simulink model "GonzalezGC21210380P3LC"  (R2024b)
settings: Solver=ode15s  StartTime=0.0  StopTime=10  MaxStep=1E-3  RelTol=1e-3
libraries: slpidlib x1
settings DataIOCC: ReturnWorkspaceOutputs=off  TimeSaveName=t
settings DebuggingCC: AlgebraicLoopMsg=none  ArtificialAlgebraicLoopMsg=none  BlockPriorityViolationMsg=error  MinStepSizeMsg=error  MaxConsecutiveZCsMsg=none  OperatingPointInterfaceChecksumMismatchMsg=none

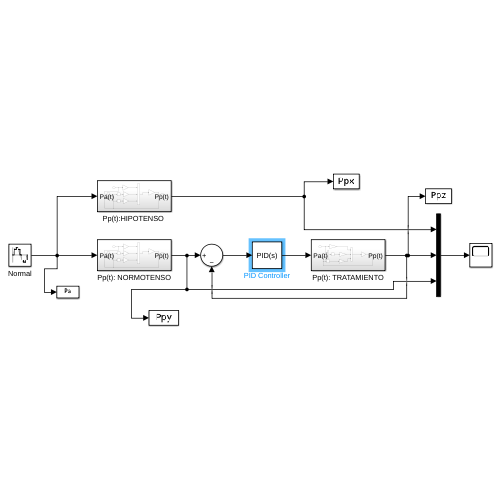
[thumbnail: Simulink's stored preview of the top-level diagram]
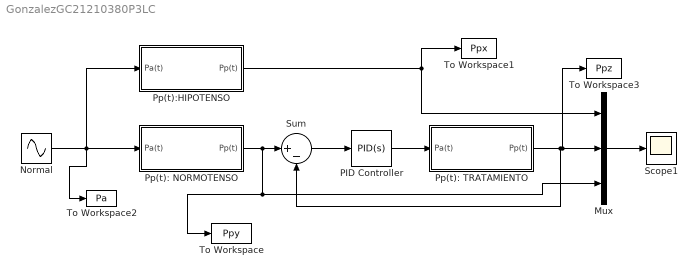
== system GonzalezGC21210380P3LC ==
  Mux : Mux  Inputs=3
  Normal : Sin  Bias=0.8  Frequency=(2*pi)*(95/60)  SampleTime=0.001
  PID Controller : slpidlib/PID Controller  Controller=PID  Form=Parallel  TimeDomain=Continuous-time  UseExternalTs=off  SampleTime=-1  IntegratorMethod=Forward Euler  FilterMethod=Forward Euler  ControllerParametersSource=internal  P=0  I=551.4981  UseKiTs=off  D=0  UseExternalDerivativeSource=off  N=100  UseFilter=on  TunerSelectOption=Transfer Function Based (PID Tuner App)  InitialConditionSource=internal  InitialConditionForIntegrator=0  InitialConditionForFilter=0  DifferentiatorICPrevScaledInput=0  ExternalReset=none  TrackingMode=off  Kt=1  LimitOutput=off  SatLimitsSource=internal  UpperSaturationLimit=inf  LowerSaturationLimit=-inf  LinearizeAsGain=on  AntiWindupMode=none  Kb=1  LimitIntegrator=off  UpperIntegratorSaturationLimit=inf  LowerIntegratorSaturationLimit=-inf  POutMin=[]  POutMax=[]  IOutMin=[]  IOutMax=[]  DOutMin=[]  DOutMax=[]  NOutMin=[]  NOutMax=[]  SumOutMin=[]  SumOutMax=[]  SaturationOutMin=[]  SaturationOutMax=[]  PParamMin=[]  PParamMax=[]  IParamMin=[]  IParamMax=[]  DParamMin=[]  DParamMax=[]  NParamMin=[]  NParamMax=[]  KbParamMin=[]  KbParamMax=[]  KtParamMin=[]  KtParamMax=[]  KbOutMin=[]  KbOutMax=[]  KtOutMin=[]  KtOutMax=[]  IntegratorOutMin=[]  IntegratorOutMax=[]  FilterOutMin=[]  FilterOutMax=[]  SumI1OutMin=[]  SumI1OutMax=[]  SumI2OutMin=[]  SumI2OutMax=[]  SumI3OutMin=[]  SumI3OutMax=[]  SumI4OutMin=[]  SumI4OutMax=[]  SumDOutMin=[]  SumDOutMax=[]  DifferentiatorOutMin=[]  DifferentiatorOutMax=[]  FilterDiffOutCoefMin=[]  FilterDiffOutCoefMax=[]  ReciprocalOutMin=[]  ReciprocalOutMax=[]  SumDenOutMin=[]  SumDenOutMax=[]  SumNumOutMin=[]  SumNumOutMax=[]  DivideOutMin=[]  DivideOutMax=[]  UdiffTsProdOutMin=[]  UdiffTsProdOutMax=[]  NTsProdOutMin=[]  NTsProdOutMax=[]  UintegralTsProdOutMin=[]  UintegralTsProdOutMax=[]  UngainTsProdOutMin=[]  UngainTsProdOutMax=[]  ClampingZeroOutDataTypeStr=Inherit: Inherit via back propagation  ClampingZeroOutMin=[]  ClampingZeroOutMax=[]  FilterDenConstantOutDataTypeStr=Inherit: Inherit via back propagation  FilterDenConstantOutMin=[]  FilterDenConstantOutMax=[]  PCopyOutDataTypeStr=Inherit: Inherit via back propagation  PCopyOutMin=[]  PCopyOutMax=[]  NCopyOutDataTypeStr=Inherit: Inherit via back propagation  NCopyOutMin=[]  NCopyOutMax=[]  IntegratorContinuousStateAttributes=''  IntegratorStateMustResolveToSignalObject=off  IntegratorRTWStateStorageClass=Auto  FilterContinuousStateAttributes=''  FilterStateMustResolveToSignalObject=off  FilterRTWStateStorageClass=Auto  ParallelPVariant=InternalParameters  IdealPVariant=Disabled  IVariant=InternalParameters  DVariant=InternalParameters  IntegratorVariant=Continuous  SatVariant=Disabled  AWVariant=Passthrough  PCopyVariant=Disabled  TRVariant=Disabled  FdbkBlocksVariant=Forward  IdealPFdbkVariant=Disabled  SatFdbkVariant=Disabled  DerivativeFilterVariant=ContFilter  NVariant=InternalParameters  NCopyVariant=Disabled  FilterICVariant=InternalICsFilter  IntegratorICVariant=InternalICs  ExternalResetVariant=Disabled  TRSumVariant=Passthrough  SumFdbkVariant=Disabled  SumVariant=Sum_PID  TsampFilterVariant=InternalTs  TsampNgainVariant=Passthrough  TsampIntegralVariant=Disabled_SignalSpec  ExternalSaturationOutDataTypeStr=Inherit: Same as second input  DerivativeSourceVariant=ErrorSignal  PreIntVariant=InternalPreInt
  Pp(t): NORMOTENSO : Subsystem
  Pp(t): TRATAMIENTO : Subsystem
  "Pp(t):HIPOTENSO " : Subsystem
  Scope1 : Scope
  Sum : Sum  Inputs=|+-
  To Workspace : ToWorkspace  VariableName=Ppy  SampleTime=-1
  To Workspace1 : ToWorkspace  VariableName=Ppx  SampleTime=-1
  To Workspace2 : ToWorkspace  VariableName=Pa  SaveFormat=Timeseries  SampleTime=-1
  To Workspace3 : ToWorkspace  VariableName=Ppz  SampleTime=-1
  wires:
  Normal/1 -> To Workspace2/1, Pp(t): NORMOTENSO/1(Pa(t)), "Pp(t):HIPOTENSO "/1(Pa(t))
  Mux/1 -> Scope1/1
  PID Controller/1 -> Pp(t): TRATAMIENTO/1(Pa(t))
  Pp(t): NORMOTENSO/1(Pp(t)) -> Mux/3, To Workspace/1, Sum/1
  Sum/1 -> PID Controller/1
  Pp(t): TRATAMIENTO/1(Pp(t)) -> Sum/2, Mux/2, To Workspace3/1
  "Pp(t):HIPOTENSO "/1(Pp(t)) -> To Workspace1/1, Mux/1

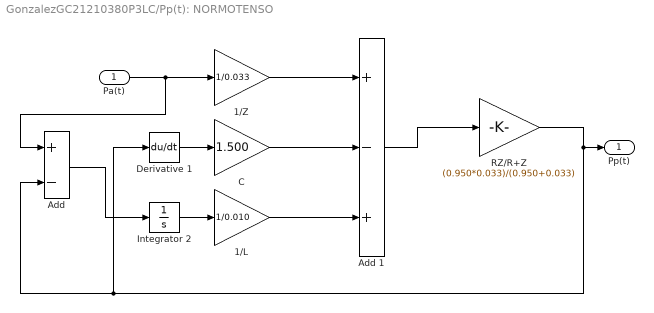
== system GonzalezGC21210380P3LC/Pp(t): NORMOTENSO ==
  Pa(t) : Inport
  1/L : Gain  Gain=1/0.010
  1/Z : Gain  Gain=1/0.033
  Add : Sum  Inputs=+-
  Add 1 : Sum  Inputs=+-+
  C : Gain  Gain=1.500
  Derivative 1 : Derivative
  Integrator 2 : Integrator
  RZ/R+Z : Gain  Gain=(0.950*0.033)/(0.950+0.033)
  Pp(t) : Outport
  wires:
  Add 1/1 -> RZ/R+Z/1
  C/1 -> Add 1/2
  RZ/R+Z/1 -> Derivative 1/1, Add/2, Pp(t)/1
  Pa(t)/1 -> Add/1, 1/Z/1
  Add/1 -> Integrator 2/1
  Integrator 2/1 -> 1/L/1
  1/L/1 -> Add 1/3
  Derivative 1/1 -> C/1
  1/Z/1 -> Add 1/1

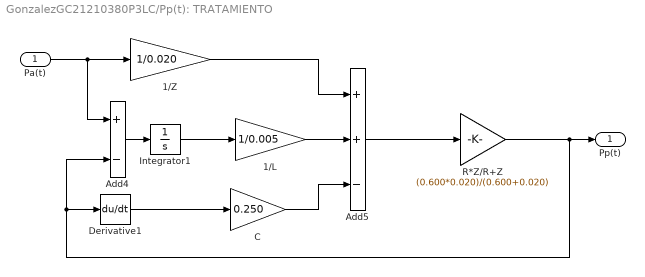
== system GonzalezGC21210380P3LC/Pp(t): TRATAMIENTO ==
  Pa(t) : Inport
  1/L : Gain  Gain=1/0.005
  1/Z : Gain  Gain=1/0.020
  Add4 : Sum  Inputs=+-
  Add5 : Sum  Inputs=++-
  C : Gain  Gain=0.250
  Derivative1 : Derivative
  Integrator1 : Integrator
  R*Z/R+Z : Gain  Gain=(0.600*0.020)/(0.600+0.020)
  Pp(t) : Outport
  wires:
  R*Z/R+Z/1 -> Derivative1/1, Add4/2, Pp(t)/1
  Pa(t)/1 -> Add4/1, 1/Z/1
  Derivative1/1 -> C/1
  1/L/1 -> Add5/2
  C/1 -> Add5/3
  Integrator1/1 -> 1/L/1
  Add4/1 -> Integrator1/1
  Add5/1 -> R*Z/R+Z/1
  1/Z/1 -> Add5/1

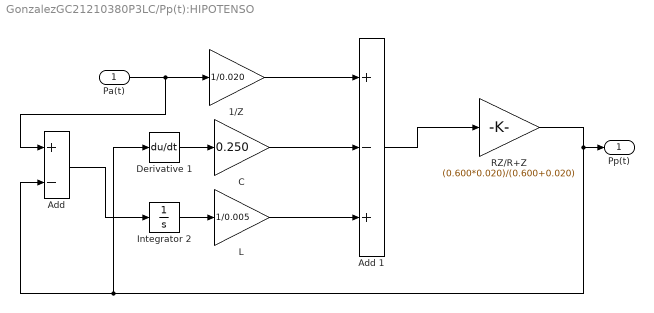
== system GonzalezGC21210380P3LC/Pp(t):HIPOTENSO  ==
  Pa(t) : Inport
  1/Z : Gain  Gain=1/0.020
  Add : Sum  Inputs=+-
  Add 1 : Sum  Inputs=+-+
  C : Gain  Gain=0.250
  Derivative 1 : Derivative
  Integrator 2 : Integrator
  L : Gain  Gain=1/0.005
  RZ/R+Z : Gain  Gain=(0.600*0.020)/(0.600+0.020)
  Pp(t) : Outport
  wires:
  Add 1/1 -> RZ/R+Z/1
  Pa(t)/1 -> Add/1, 1/Z/1
  1/Z/1 -> Add 1/1
  C/1 -> Add 1/2
  L/1 -> Add 1/3
  Derivative 1/1 -> C/1
  Integrator 2/1 -> L/1
  RZ/R+Z/1 -> Derivative 1/1, Add/2, Pp(t)/1
  Add/1 -> Integrator 2/1
